simulink model "IndustrialMicrogrid"  (R2025a)
settings: Solver=FixedStepAuto  StartTime=0.0  StopTime=8  FixedStep=Ts  RelTol=1e-3
PostLoadFcn:
  | IndustrialMicrogridInputData
  | GfmGridFormingConverterInputParameters
model workspace (MAT data in the model file):
  caseNum = 2
undefined symbols (not defined in the file): base, BESS, DiscIntNeverNeededParam, grid, Grid, gridInverter, machine, microgrid, PV, PVInverter, PVTransformer, scrFactorRg, scrFactorXg, transformer, Transition_and_Dispatch_ControlModeType, Ts
libraries: ee_lib x126, fl_lib x91, eeGeneralControl x73, nesl_utility x50, nesl_utility_internal x46, simulink x30, eeTransforms x11, eeSinusoidalMeasurementV2 x5, eeTotalHarmonicDistorsion x4, slpidlib x3, simulink_extras x2, eePowerMeasurement x2
(part 2 of 12)

== system IndustrialMicrogrid/MG2 Main Grid ==
  Electrical Reference1 : fl_lib/Electrical/Electrical Elements/Electrical Reference
  Main Grid Frequency : Constant  Value=grid.frequency  SampleTime=-1
  Programmable Voltage Source (Three-Phase)2 : ee_lib/Sources/Programmable Voltage Source (Three-Phase)  magnitude_type=ee.enum.timechanging.constant  vline_rms=grid.voltageSource V  magn_ramp=1 V/s  magn_step=1 V  magn_modu_magn=1 V  magn_modu_freq=1 Hz  magn_t1=1 s  magn_t2=2 s  frequency_type=ee.enum.timechanging.external  freq=50 Hz  freq_ramp=1 Hz/s  freq_step=1 Hz  freq_modu_magn=1 Hz  freq_modu_freq=1 Hz  freq_t1=1 s  freq_t2=2 s  phase_type=ee.enum.timechanging.constant  shift=0 deg  phase_ramp=1 deg/s  phase_step=1 deg  phase_modu_magn=1 deg  phase_modu_freq=1 Hz  phase_t1=1 s  phase_t2=2 s  impedance_option=1  SShortCircuit=100e6 A*V  XR=15  R=0.01 Ohm  L=3.97e-4*0.1 H  G_parasitic=1e-6 1/Ohm  harmonic_option=0  harmonic_orders=[5, 7, 11, 13]  harmonic_ratios=[.1, .1, .1, .1]  harmonic_shifts=[0, 0, 0, 0] deg  harmonic_sequences=[1, 1, 1, 1]  harmonic_t1=-inf s  harmonic_t2=inf s  I_specify=on  I_priority=None  I=[0, 0, 0] A  I_nominal_specify=off  I_nominal_value=1  I_nominal_unit=A  V_specify=on  V_priority=None  V=[0, 0, 0] V  V_nominal_specify=off  V_nominal_value=1  V_nominal_unit=V
      settings: InternalSimscapePortConfiguration="{\"Bottom\":[],\"Left\":[{\"id\":\"ext_freq\",\"label\":\"F\",\"type\":\"input\"},{\"id\":\"n\",\"label\":\"n\",\"type\":\"foundation.electrical.electrical\"}],\"Right\":[{\"id\":\"N\",\"label\":\"~\",\"type\":\"foundation.electrical.three_phase\"}],\"Top\":[]}"
  Simulink-PS Converter : nesl_utility_internal/Simulink-PS Converter  PhysicalDomain=network_engine_domain  SubClassName=ps_input  LeftPortType=input  RightPortType=output  PseudoPeriodic=off  Frequencies=[]  NoiseDistribution=none  NoiseParameters=[]  Unit=1  AffineConversion=off  FilteringAndDerivatives=provide  SimscapeFilterOrder=1  InputFilterTimeConstant=0.001  UdotUserProvided=0
  Source impedance and Line X/R=18.8 : ee_lib/Passive/RLC Assemblies/RLC (Three-Phase)  port_option=ee.enum.threePhasePort.composite  component_structure=ee.enum.rlc.structure.SeriesRL  R=grid.rMV Ohm  L=grid.lMV1 H  C=1e-6 F  R_parasitic=1e-6 Ohm  G_parasitic=1e-6 1/Ohm  IL_specify=on  IL_priority=None  IL=[0, 0, 0] A  IL_nominal_specify=off  IL_nominal_value=1  IL_nominal_unit=A  VC_specify=off  VC_priority=High  VC=[0, 0, 0] V  VC_nominal_specify=off  VC_nominal_value=1  VC_nominal_unit=V
      settings: InternalSimscapePortConfiguration="{\"Bottom\":[],\"Left\":[{\"id\":\"N1\",\"label\":\"~1\",\"type\":\"foundation.electrical.three_phase\"}],\"Right\":[{\"id\":\"N2\",\"label\":\"~2\",\"type\":\"foundation.electrical.three_phase\"}],\"Top\":[]}"
  ref : PMIOPort  Side=Left
  ~ : PMIOPort  Port=2  Side=Right
  wires:
  Main Grid Frequency/1 -> Simulink-PS Converter/1
  connections:
  ref/RConn1 -- Electrical Reference1/LConn1 -- Programmable Voltage Source (Three-Phase)2/LConn2
  Source impedance and Line X/R=18.8/LConn1 -- Programmable Voltage Source (Three-Phase)2/RConn1
  Source impedance and Line X/R=18.8/RConn1 -- ~/RConn1
  Simulink-PS Converter/RConn1 -- Programmable Voltage Source (Three-Phase)2/LConn1

== system IndustrialMicrogrid/MG2 PV Plant ==
  (500KWp PV) : Subsystem
      settings: PortSchema="{\"entries\":[{\"content\":{\"sides\":[{\"content\":{\"connectorIds\":[\"Out1\",\"In1\",\"LConn1\"]},\"type\":\"ConnectorPlacement.EquallySpacedRectSide\",\"uuid\":\"7b0e71bf-88d0-4fd9-b424-51733315768d\"},{\"content\":{\"side\":\"RIGHT\"},\"type\":\"ConnectorPlacement.EquallySpacedRectSide\",\"uuid\":\"454a206f-9a61-4ac7-86a8-f6508f61436e\"},{\"content\":{\"side\":\"TOP\"},\"type\":\"ConnectorPlacement.EquallySpacedRectSide\",\"uuid\":\"cf982e1c-b164-4d0a-abcb-f158cc5498a1\"}]},\"type\":\"ConnectorPlacement.EquallySpacedConnector\",\"uuid\":\"7d6089e9-e0b0-4b95-be20-3597ac4fefae\"}],\"packageUris\":[\"http://schema.mathworks.com/mf0/Connector/R2020b\"],\"version\":\"1.0\"}"
  4.16 kV/ 13.8 kV2 : ee_lib/Passive/Transformers/Two-Winding Transformer (Three-Phase)  SRated=PVTransformer.VA A*V  FRated=grid.frequency Hz  Winding1Connection=ee.enum.windingconnection.delta1  VRated1=PVTransformer.hv V  Winding2Connection=ee.enum.windingconnection.Yn  VRated2=PVTransformer.lv V  CoreType=ee.enum.coretype.threelimb  pu_Rw1=PVTransformer.windingResistance*1/2  pu_Rw2=PVTransformer.windingResistance*1/2  leakage_reactance_option=ee.enum.transformer_leakage.include  pu_Xl1=PVTransformer.windingLekageReactance*1/2  pu_Xl2=PVTransformer.windingLekageReactance*1/2  magnetizing_resistance_option=ee.enum.transformer_magnetizingResistance.exclude  pu_Rm=500  magnetizing_reactance_option=ee.enum.transformer_magnetizingReactance.exclude  saturation_option=ee.enum.transformer_saturation.exclude  pu_Xm=500  current_data=[0, .002, 1, 2]  magnetic_flux_data=[0, 1.2, 1.5, 1.51]  pu_X0=PVTransformer.zeroSequenceReactance*1.5  i1_specify=off  i1_priority=None  i1=[0, 0, 0] A  i1_nominal_specify=off  i1_nominal_value=1  i1_nominal_unit=A  i2_specify=off  i2_priority=None  i2=[0, 0, 0] A  i2_nominal_specify=off  i2_nominal_value=1  i2_nominal_unit=A  phi_specify=off  phi_priority=None  phi=[0, 0, 0]  phi_nominal_specify=off  phi_nominal_value=1  phi_nominal_unit=1  power_dissipated_specify=off  power_dissipated_priority=None  power_dissipated=0 W  power_dissipated_nominal_specify=off  power_dissipated_nominal_value=1  power_dissipated_nominal_unit=W
      settings: InternalSimscapePortConfiguration="{\"Bottom\":[],\"Left\":[{\"id\":\"N1\",\"label\":\"~1\",\"type\":\"foundation.electrical.three_phase\"}],\"Right\":[{\"id\":\"N2\",\"label\":\"~2\",\"type\":\"foundation.electrical.three_phase\"},{\"id\":\"n2\",\"label\":\"n2\",\"type\":\"foundation.electrical.electrical\"}],\"Top\":[]}"
  Bus Creator : BusCreator  Inputs=2
  Bus Selector : BusSelector  OutputSignals=Vmag
  Circuit Breaker : Subsystem
  Current and Voltage Sensor (Three-Phase)1 : ee_lib/Sensors & Transducers/Current and Voltage Sensor (Three-Phase)  vMeasurementType=ee.enum.vmeasurement.lg  outputUnit=ee.enum.unit.pu  SRated=PV.MVABaseNew A*V  VRated=PV.kVBaseNew V  I_specify=off  I_priority=None  I=[0, 0, 0] A  I_nominal_specify=off  I_nominal_value=1  I_nominal_unit=A  V_specify=off  V_priority=None  V=[0, 0, 0] V  V_nominal_specify=off  V_nominal_value=1  V_nominal_unit=V
      settings: InternalSimscapePortConfiguration="{\"Bottom\":[],\"Left\":[{\"id\":\"N1\",\"label\":\"~1\",\"type\":\"foundation.electrical.three_phase\"}],\"Right\":[{\"id\":\"V_output\",\"label\":\"V\",\"type\":\"output\"},{\"id\":\"I_output\",\"label\":\"I\",\"type\":\"output\"},{\"id\":\"N2\",\"label\":\"~2\",\"type\":\"foundation.electrical.three_phase\"}],\"Top\":[]}"
  Electrical Reference8 : fl_lib/Electrical/Electrical Elements/Electrical Reference
  PLL & Measurements2 : Subsystem
  PS-Simulink Converter1 : nesl_utility/PS-Simulink Converter  PhysicalDomain=network_engine_domain  SubClassName=ps_output  LeftPortType=input  RightPortType=output  PseudoPeriodic=off  Frequencies=[]  VectorFormat=inherit  Unit=inherit  AffineConversion=off
  PS-Simulink Converter2 : nesl_utility/PS-Simulink Converter  PhysicalDomain=network_engine_domain  SubClassName=ps_output  LeftPortType=input  RightPortType=output  PseudoPeriodic=off  Frequencies=[]  VectorFormat=inherit  Unit=inherit  AffineConversion=off
  Step : Step  Time=microgrid.controller2PVBrk  Before=1  After=0  SampleTime=2*Ts
  Terminator : Terminator
  ~ : PMIOPort  Side=Left
  mPV : Outport
  wires:
  (500KWp PV)/1(PV) -> Bus Creator/1  "PV"
  PS-Simulink Converter1/1 -> Terminator/1
  Bus Creator/1 -> mPV/1  "mPV"
  PLL & Measurements2/1(Vbus) -> (500KWp PV)/1(Vbus), Bus Selector/1
  PS-Simulink Converter2/1 -> PLL & Measurements2/1(V)
  Bus Selector/1 -> Bus Creator/2  "<Vmag>"
  Step/1 -> Circuit Breaker/1(BRK)
  connections:
  Current and Voltage Sensor (Three-Phase)1/RConn3 -- 4.16 kV/ 13.8 kV2/RConn1
  Current and Voltage Sensor (Three-Phase)1/RConn2 -- PS-Simulink Converter1/LConn1
  4.16 kV/ 13.8 kV2/RConn2 -- Electrical Reference8/LConn1
  Current and Voltage Sensor (Three-Phase)1/RConn1 -- PS-Simulink Converter2/LConn1
  4.16 kV/ 13.8 kV2/LConn1 -- ~/RConn1
  Circuit Breaker/RConn1 -- Current and Voltage Sensor (Three-Phase)1/LConn1
  Circuit Breaker/LConn1 -- (500KWp PV)/LConn1

== system IndustrialMicrogrid/MG2 Power Center ==
  Bus Element In1 : Inport  PortName=ControlRoom  Element=brk2
  Bus Element In2 : Inport  PortName=ControlRoom  Element=dieselBrk
  Bus Element In4 : Inport  PortName=ControlRoom  Element=brk3
  Bus Element In3 : Inport  PortName=ControlRoom  Element=brk1
  BusElementIn : Inport  PortName=ControlRoom  Element=brk4
  Circuit Breaker : Subsystem
  Circuit Breaker1 : Subsystem
      settings: PortSchema="{\"entries\":[{\"content\":{\"sides\":[{\"content\":{\"connectorIds\":[\"LConn1\",\"In1\"]},\"type\":\"ConnectorPlacement.EquallySpacedRectSide\",\"uuid\":\"61e5b689-674d-42bf-9486-b78d237e4dc5\"},{\"content\":{\"connectorIds\":[\"RConn1\"],\"side\":\"RIGHT\"},\"type\":\"ConnectorPlacement.EquallySpacedRectSide\",\"uuid\":\"9e681376-db09-4bc3-bcf5-1ab917668327\"},{\"content\":{\"side\":\"TOP\"},\"type\":\"ConnectorPlacement.EquallySpacedRectSide\",\"uuid\":\"9b4580d8-22f1-4808-acc6-ee968907ce8f\"},{\"content\":{\"side\":\"BOTTOM\"},\"type\":\"ConnectorPlacement.EquallySpacedRectSide\",\"uuid\":\"ecc9f1e9-f021-446f-9399-19e509bfd837\"}]},\"type\":\"ConnectorPlacement.EquallySpacedConnector\",\"uuid\":\"3c8ab3c7-5612-487b-b971-89e63217e257\"}],\"packageUris\":[\"http://schema.mathworks.com/mf0/Connector/R2020b\"],\"version\":\"1.0\"}"
  Circuit Breaker3 : Subsystem
  Circuit Breaker4 : Subsystem
  Diesel Generator : Subsystem
      mask Display: image('$imagefile'); % Use "Edit Image" on toolstrip to change.
  Diesel Measurements : Subsystem
  Fault (Three-Phase) : ee_lib/Utilities/Fault (Three-Phase)  fault_type_option=11  R_pn_fault=3 Ohm  R_ng_fault=3 Ohm  exposemeasurement=ee.enum.exposemeasurement.hidden  enable_external_fault=ee.enum.external_fault.hidden  fault_threshold=0.5  fault_condition=1  fault_resettable=0  enable_temporal_fault=1  fault_start_time=microgrid.controller2PowerCenterFault s  fault_duration=0.3 s  G_parasitic=1e-6 1/Ohm
      settings: InternalSimscapePortConfiguration="{\"Bottom\":[],\"Left\":[{\"id\":\"N\",\"label\":\"~\",\"type\":\"foundation.electrical.three_phase\"}],\"Right\":[],\"Top\":[]}"
  Line X/R=1.44 1 : ee_lib/Passive/RLC Assemblies/RLC (Three-Phase)  port_option=ee.enum.threePhasePort.composite  component_structure=ee.enum.rlc.structure.SeriesRL  R=microgrid.rLine*0.2 Ohm  L=microgrid.lLine*0.2 H  C=1 F  R_parasitic=1e-6 Ohm  G_parasitic=1e-5 1/Ohm  IL_specify=on  IL_priority=None  IL=[0, 0, 0] A  IL_nominal_specify=off  IL_nominal_value=1  IL_nominal_unit=A  VC_specify=on  VC_priority=High  VC=[0, 0, 0] V  VC_nominal_specify=off  VC_nominal_value=1  VC_nominal_unit=V
      settings: InternalSimscapePortConfiguration="{\"Bottom\":[],\"Left\":[{\"id\":\"N1\",\"label\":\"~1\",\"type\":\"foundation.electrical.three_phase\"}],\"Right\":[{\"id\":\"N2\",\"label\":\"~2\",\"type\":\"foundation.electrical.three_phase\"}],\"Top\":[]}"
  Line X/R=1.44 2 : ee_lib/Passive/RLC Assemblies/RLC (Three-Phase)  port_option=ee.enum.threePhasePort.composite  component_structure=ee.enum.rlc.structure.SeriesRL  R=microgrid.rLine*0.3 Ohm  L=microgrid.lLine*0.3 H  C=1 F  R_parasitic=1e-6 Ohm  G_parasitic=1e-5 1/Ohm  IL_specify=on  IL_priority=None  IL=[0, 0, 0] A  IL_nominal_specify=off  IL_nominal_value=1  IL_nominal_unit=A  VC_specify=on  VC_priority=High  VC=[0, 0, 0] V  VC_nominal_specify=off  VC_nominal_value=1  VC_nominal_unit=V
      settings: InternalSimscapePortConfiguration="{\"Bottom\":[],\"Left\":[{\"id\":\"N1\",\"label\":\"~1\",\"type\":\"foundation.electrical.three_phase\"}],\"Right\":[{\"id\":\"N2\",\"label\":\"~2\",\"type\":\"foundation.electrical.three_phase\"}],\"Top\":[]}"
  Line X/R=1.44 3 : ee_lib/Passive/RLC Assemblies/RLC (Three-Phase)  port_option=ee.enum.threePhasePort.composite  component_structure=ee.enum.rlc.structure.SeriesRL  R=microgrid.rLine*0.2 Ohm  L=microgrid.lLine*0.2 H  C=1 F  R_parasitic=1e-6 Ohm  G_parasitic=1e-5 1/Ohm  IL_specify=on  IL_priority=None  IL=[0, 0, 0] A  IL_nominal_specify=off  IL_nominal_value=1  IL_nominal_unit=A  VC_specify=on  VC_priority=High  VC=[0, 0, 0] V  VC_nominal_specify=off  VC_nominal_value=1  VC_nominal_unit=V
      settings: InternalSimscapePortConfiguration="{\"Bottom\":[],\"Left\":[{\"id\":\"N1\",\"label\":\"~1\",\"type\":\"foundation.electrical.three_phase\"}],\"Right\":[{\"id\":\"N2\",\"label\":\"~2\",\"type\":\"foundation.electrical.three_phase\"}],\"Top\":[]}"
  Low-Pass Filter (Discrete or Continuous) : eeGeneralControl/Low-Pass Filter (Discrete or Continuous)  K=1  T=0.1  B=inf  A=-inf  init_option=Inherited from block input  x0=0  Ts=Ts
  Low-Pass Filter (Discrete or Continuous)1 : eeGeneralControl/Low-Pass Filter (Discrete or Continuous)  K=1  T=0.1  B=inf  A=-inf  init_option=Inherited from block input  x0=0  Ts=Ts
  PS-Simulink Converter8 : nesl_utility_internal/PS-Simulink Converter  PhysicalDomain=network_engine_domain  SubClassName=ps_output  LeftPortType=input  RightPortType=output  PseudoPeriodic=off  Frequencies=[]  VectorFormat=1-D array  Unit=MW  AffineConversion=off
  PS-Simulink Converter9 : nesl_utility_internal/PS-Simulink Converter  PhysicalDomain=network_engine_domain  SubClassName=ps_output  LeftPortType=input  RightPortType=output  PseudoPeriodic=off  Frequencies=[]  VectorFormat=1-D array  Unit=MV*A  AffineConversion=off
  Power Sensor (Three-Phase)2 : ee_lib/Sensors & Transducers/Power Sensor (Three-Phase)  load_type=ee.enum.passive.type_balanced.balanced  f0=60 Hz  config=ee.enum.with_neutral.no  rho=1
      settings: InternalSimscapePortConfiguration="{\"Bottom\":[],\"Left\":[{\"id\":\"N1\",\"label\":\"~1\",\"type\":\"foundation.electrical.three_phase\"}],\"Right\":[{\"id\":\"N2\",\"label\":\"~2\",\"type\":\"foundation.electrical.three_phase\"}],\"Top\":[{\"id\":\"Pm\",\"label\":\"P\",\"type\":\"output\"},{\"id\":\"Qm\",\"label\":\"Q\",\"type\":\"output\"}]}"
  Transformer and Disconnectors : Subsystem
      mask Display: image('$imagefile'); % Use "Edit Image" on toolstrip to change.
  Two-Winding Transformer (Three-Phase)1 : ee_lib/Passive/Transformers/Two-Winding Transformer (Three-Phase)  SRated=microgrid.powerCenterTransformerRating A*V  FRated=microgrid.frequency Hz  Winding1Connection=ee.enum.windingconnection.Y  VRated1=microgrid.powerCenterTransformerPrimaryVoltage V  Winding2Connection=ee.enum.windingconnection.Y  VRated2=microgrid.powerCenterTransformerSecondaryVoltage V  CoreType=ee.enum.coretype.threelimb  pu_Rw1=microgrid.powerCenterPrimaryresistance  pu_Rw2=microgrid.powerCenterPrimaryreactance  leakage_reactance_option=ee.enum.transformer_leakage.include  pu_Xl1=microgrid.powerCenterSecondaryresistance  pu_Xl2=microgrid.powerCenterSecondaryreactance  magnetizing_resistance_option=ee.enum.transformer_magnetizingResistance.include  pu_Rm=500  magnetizing_reactance_option=ee.enum.transformer_magnetizingReactance.include  saturation_option=ee.enum.transformer_saturation.exclude  pu_Xm=500  current_data=[0, .002, 1, 2]  magnetic_flux_data=[0, 1.2, 1.5, 1.51]  pu_X0=0.5  i1_specify=on  i1_priority=None  i1=[0, 0, 0] A  i1_nominal_specify=off  i1_nominal_value=1  i1_nominal_unit=A  i2_specify=on  i2_priority=None  i2=[0, 0, 0] A  i2_nominal_specify=off  i2_nominal_value=1  i2_nominal_unit=A  phi_specify=off  phi_priority=None  phi=[0, 0, 0]  phi_nominal_specify=off  phi_nominal_value=1  phi_nominal_unit=1  power_dissipated_specify=off  power_dissipated_priority=None  power_dissipated=0 W  power_dissipated_nominal_specify=off  power_dissipated_nominal_value=1  power_dissipated_nominal_unit=W
      settings: InternalSimscapePortConfiguration="{\"Bottom\":[],\"Left\":[{\"id\":\"N1\",\"label\":\"~1\",\"type\":\"foundation.electrical.three_phase\"}],\"Right\":[{\"id\":\"N2\",\"label\":\"~2\",\"type\":\"foundation.electrical.three_phase\"}],\"Top\":[]}"
  Conn2 : PMIOPort  Side=Left
  ~ a : PMIOPort  Port=2  Side=Left
  " ~ " : PMIOPort  Port=3  Side=Right
  Out Bus Element2 : Outport  PortName=mPowerCentre  Element=tieline.activepower
  Out Bus Element3 : Outport  PortName=mPowerCentre  Element=tieline.reactivepower
  Out Bus Element1 : Outport  PortName=mPowerCentre  Element=diesel
  wires:
  Bus Element In3/1 -> Circuit Breaker/1(BRK)
  PS-Simulink Converter8/1 -> Low-Pass Filter (Discrete or Continuous)/1
  Low-Pass Filter (Discrete or Continuous)1/1 -> Out Bus Element3/1
  PS-Simulink Converter9/1 -> Low-Pass Filter (Discrete or Continuous)1/1
  Low-Pass Filter (Discrete or Continuous)/1 -> Out Bus Element2/1
  Bus Element In4/1 -> Circuit Breaker3/1(BRK)
  Bus Element In2/1 -> Circuit Breaker4/1(BRK)
  Diesel Measurements/1(mdiesel) -> Out Bus Element1/1  "diesel"
  Bus Element In1/1 -> Circuit Breaker1/1(BRK)
  BusElementIn/1 -> Transformer and Disconnectors/1(BRK)
  connections:
  Line X/R=1.44 1/RConn1 -- ~ a/RConn1 -- Fault (Three-Phase)/LConn1
  Line X/R=1.44 3/RConn1 -- " ~ "/RConn1
  Circuit Breaker/RConn1 -- Circuit Breaker3/LConn1 -- Circuit Breaker1/LConn1
  Line X/R=1.44 2/LConn1 -- Conn2/RConn1
  Diesel Generator/RConn1 -- Transformer and Disconnectors/LConn1
  Two-Winding Transformer (Three-Phase)1/RConn1 -- Circuit Breaker4/RConn1 -- Line X/R=1.44 3/LConn1
  Transformer and Disconnectors/RConn1 -- Diesel Measurements/LConn1
  Circuit Breaker3/RConn1 -- Line X/R=1.44 1/LConn1
  PS-Simulink Converter9/LConn1 -- Power Sensor (Three-Phase)2/LConn3
  PS-Simulink Converter8/LConn1 -- Power Sensor (Three-Phase)2/LConn2
  Power Sensor (Three-Phase)2/LConn1 -- Line X/R=1.44 2/RConn1
  Circuit Breaker/LConn1 -- Power Sensor (Three-Phase)2/RConn1
  Circuit Breaker1/RConn1 -- Two-Winding Transformer (Three-Phase)1/LConn1
  Circuit Breaker4/LConn1 -- Diesel Measurements/RConn1

== system IndustrialMicrogrid/MG2 Primary Substation ==
  ControlRoom : Inport
  BESS and Controller : Subsystem
  Bus Selector : BusSelector  OutputSignals=Substation.brk
  Circuit Breaker : Subsystem
  Microgrid Controller : Subsystem  mask{resynchronization=on, plannedIslanding=on, blackStart=on, kpPLL=microgrid.KpPLLController2, kiPLL=microgrid.KiPLLController2, frequencyPLL=grid.frequency, sampleTimePLL=Ts, pUpperLimit=1.2, pLowerLimit=-1.2, qUpperLimit=1.2, qLowerLimit=-1.2, gridFrequency=grid.frequency, resyncDelay=microgrid.resynchDelay, kpVoltage=microgrid.KpVolResynch2, kiVoltage=microgrid.KiVolResynch2, voltageThreshold=microgrid.voltageThreshold, voltageDroop=microgrid.KDroop, kpFrequency=microgrid.KpFreResynch2, kiFrequency=microgrid.KiFreResynch2, frequencyThreshold=microgrid.frequencyThreshold, kpAngle=microgrid.KpAngResynch2, kiAngle=microgrid.KiAngResynch2, angleThreshold=microgrid.angleThreshold, plannedIslandingDelay=microgrid.plannedIslandDelay, kpActive=microgrid.KpPPlannedIsland2, kiActive=microgrid.KiPPlannedIsland2, activeThreshold=microgrid.zeroActivePowerThreshold, kpReactive=microgrid.KpQPlannedIsland2, kiReactive=microgrid.KiQPlannedIsland2, reactiveThreshold=microgrid.zeroReactivePowerThreshold, blackStartTime=microgrid.controller2BlackStartDelay, blackStartFrequency=60, level1=microgrid.controller2BlackStartVoltageLevel1, level2=microgrid.controller2BlackStartVoltageLevel2, level3=microgrid.controller2BlackStartVoltageLevel3, delay1=microgrid.controller2BlackStartDelayLevel1, delay2=microgrid.controller2BlackStartDelayLevel2, delay3=microgrid.controller2BlackStartDelayLevel3, upperVoltagelimit=1.1, lowerVoltageLimit=0.9, upperFrequencyLimit=60.6, lowerFrequencyLimit=59.4}
      mask prompts: plannedIslanding "Planned Islanding"; blackStart "Black Start"; kpPLL "Proportional Gain"; kiPLL "Integral Gain"; frequencyPLL "Grid Frequency in Hz"; sampleTimePLL "Sample Time in sec"; pUpperLimit "Upper Limit in pu"; pLowerLimit "Lower Limit in pu"; qUpperLimit "Upper Limit in pu"; qLowerLimit "Lower Limit in pu"; gridFrequency "Grid Frequency in Hz"; resyncDelay "Delay in sec"; kpVoltage "Proportional Gain"; kiVoltage "Voltage Integral Gain"; voltageThreshold "Threshold"; voltageDroop "Reactive Power Droop"; kpFrequency "Proportional Gain"; kiFrequency "Integral Gain"; frequencyThreshold "Threshold"; kpAngle "Proportional Gain"; kiAngle "Integral Gain"; angleThreshold "Threshold"; plannedIslandingDelay "Delay in sec"; kpActive "Proportional Gain"; kiActive "Integral Gain"; activeThreshold "Threshold"; kpReactive "Proportional Gain"; kiReactive "Integral Gain"; reactiveThreshold "Threshold"; blackStartTime "Black Start Time in sec"; blackStartFrequency "Reference Frequency in Hz"; level1 "Level 1 in pu"; level2 "Level 2 in pu"; level3 "Level 3 in pu"; delay1 "Delay 1 in sec"; delay2 "Delay2 in sec"; delay3 "Delay3 in sec"; upperVoltagelimit "Maximum Voltage in pu"; lowerVoltageLimit "Minimum Voltage in pu"; upperFrequencyLimit "Maximum frequency in Hz"; lowerFrequencyLimit "Minimum Frequency in Hz"
      mask init: same as IndustrialMicrogrid/MG1 Primary Substation/Microgrid Controller
      mask Callback resynchronization:
      | plannedIslandingBlock = [gcb,'/','Microgrid Control Functions','/','Planned Islanding'];
      | resynchBlock = [gcb,'/','Microgrid Control Functions','/','Resynchronization'];
      | blackStartBlock = [gcb,'/','Microgrid Control Functions','/','Black Start'];
      | block = {resynchBlock,plannedIslandingBlock,blackStartBlock};
      | blockEnable = {get_param(gcb,'resynchronization'),get_param(gcb,'plannedIslanding'),get_param(gcb,'blackStart')};
      | parameterIdx = {12:23,24:30,31:38};
      | % Set the 'MaskVisibilities' property for each parameters
      | cArray=cell(1,42);
      | cArray(:)={'on'};
      | for blockIdx = 1:length(block)
      |     if strcmp(blockEnable{blockIdx},'on')
      |         cArray(parameterIdx{blockIdx}) = {'on'};
      |     else
      |         cArray(parameterIdx{blockIdx}) = {'off'};
      |     end
      | end
      | set_param(gcb,'MaskVisibilities',cArray);
      mask Callback plannedIslanding:
      | plannedIslandingBlock = [gcb,'/','Microgrid Control Functions','/','Planned Islanding'];
      | resynchBlock = [gcb,'/','Microgrid Control Functions','/','Resynchronization'];
      | blackStartBlock = [gcb,'/','Microgrid Control Functions','/','Black Start'];
      | block = {resynchBlock,plannedIslandingBlock,blackStartBlock};
      | blockEnable = {get_param(gcb,'resynchronization'),get_param(gcb,'plannedIslanding'),get_param(gcb,'blackStart')};
      | parameterIdx = {12:23,24:30,31:38};
      | % Set the 'MaskVisibilities' property for each parameters
      | cArray=cell(1,42);
      | cArray(:)={'on'};
      | for blockIdx = 1:length(block)
      |     if strcmp(blockEnable{blockIdx},'on')
      |         cArray(parameterIdx{blockIdx}) = {'on'};
      |     else
      |         cArray(parameterIdx{blockIdx}) = {'off'};
      |     end
      | end
      | set_param(gcb,'MaskVisibilities',cArray);
      mask Callback blackStart:
      | plannedIslandingBlock = [gcb,'/','Microgrid Control Functions','/','Planned Islanding'];
      | resynchBlock = [gcb,'/','Microgrid Control Functions','/','Resynchronization'];
      | blackStartBlock = [gcb,'/','Microgrid Control Functions','/','Black Start'];
      | block = {resynchBlock,plannedIslandingBlock,blackStartBlock};
      | blockEnable = {get_param(gcb,'resynchronization'),get_param(gcb,'plannedIslanding'),get_param(gcb,'blackStart')};
      | parameterIdx = {12:23,24:30,31:38};
      | % Set the 'MaskVisibilities' property for each parameters
      | cArray=cell(1,42);
      | cArray(:)={'on'};
      | for blockIdx = 1:length(block)
      |     if strcmp(blockEnable{blockIdx},'on')
      |         cArray(parameterIdx{blockIdx}) = {'on'};
      |     else
      |         cArray(parameterIdx{blockIdx}) = {'off'};
      |     end
      | end
      | set_param(gcb,'MaskVisibilities',cArray);
      mask DialogControl ParameterGroupVar Prompt: Microgrid control functions
      mask DialogControl Container22 Prompt: PLL
      mask DialogControl Container25 Prompt: General
      mask DialogControl Container23 Prompt: Reference Generation
      mask DialogControl Container27 Prompt: Active Power
      mask DialogControl Container28 Prompt: Reactive Power
      mask DialogControl Container3 Prompt: Resynchronization
      mask DialogControl Container15 Prompt: General
      mask DialogControl Container9 Prompt: Voltage
      mask DialogControl Container10 Prompt: Frequency
      mask DialogControl Container11 Prompt: Angle
      mask DialogControl Container8 Prompt: Planned Islanding
      mask DialogControl Container16 Prompt: General
      mask DialogControl Container13 Prompt: Active Power
      mask DialogControl Container14 Prompt: Reactive Power
      mask DialogControl Container17 Prompt: Black Start
      mask DialogControl Container19 Prompt: General
      mask DialogControl Container20 Prompt: Voltage Levels
      mask DialogControl Container21 Prompt: Time Delays
      mask DialogControl Container261 Prompt: Power Quality Metrics
      mask Display: image('$imagefile'); % Use "Edit Image" on toolstrip to change.
  PCC Measurements and PCC Breaker : Subsystem
      settings: PortSchema="{\"entries\":[{\"content\":{\"sides\":[{\"content\":{\"connectorIds\":[\"In1\",\"LConn1\"]},\"type\":\"ConnectorPlacement.EquallySpacedRectSide\",\"uuid\":\"8d1da80d-0887-44e0-a470-a36b233902dd\"},{\"content\":{\"connectorIds\":[\"RConn1\",\"Out1\"],\"side\":\"RIGHT\"},\"type\":\"ConnectorPlacement.EquallySpacedRectSide\",\"uuid\":\"69fb492f-8375-4103-b8b2-15eabe039e82\"},{\"content\":{\"side\":\"TOP\"},\"type\":\"ConnectorPlacement.EquallySpacedRectSide\",\"uuid\":\"e2b1d5d4-ee63-40b0-8f64-d550ce16e67b\"}]},\"type\":\"ConnectorPlacement.EquallySpacedConnector\",\"uuid\":\"58949bb1-e57a-47d5-a7ba-dffc622c6db7\"}],\"packageUris\":[\"http://schema.mathworks.com/mf0/Connector/R2020b\"],\"version\":\"1.0\"}"
      mask Display: image('$imagefile'); % Use "Edit Image" on toolstrip to change.
  Transformer and Disconnectors : Subsystem
      mask Display: image('$imagefile'); % Use "Edit Image" on toolstrip to change.
  ~ : PMIOPort  Side=Left
  "~ " : PMIOPort  Port=2  Side=Right
  Out Bus Element : Outport  PortName=MG2  Element=mBESS
  Out Bus Element1 : Outport  PortName=MG2  Element=mPCC
  Out Bus Element2 : Outport  PortName=MG2  Element=MGController
  wires:
  ControlRoom/1 -> BESS and Controller/1(CntrlRmIN), Bus Selector/1, Microgrid Controller/1(CtrlRm)
  Microgrid Controller/3(PQRef) -> BESS and Controller/4(PQref)
  Microgrid Controller/2(FRef) -> BESS and Controller/3(f0)
  Microgrid Controller/1(VRef) -> BESS and Controller/2(Vref)
  Microgrid Controller/5(PCC BRK) -> PCC Measurements and PCC Breaker/1(cBreaker)
  PCC Measurements and PCC Breaker/1(" mPCC") -> Out Bus Element1/1, Microgrid Controller/2(mPCC)  "mPCC"
  BESS and Controller/1(mBESS) -> Out Bus Element/1  "BESS2"
  Microgrid Controller/4(MGController) -> Out Bus Element2/1  "MGController"
  Bus Selector/1 -> Circuit Breaker/1(BRK)  "<brk>"
  connections:
  ~/RConn1 -- Transformer and Disconnectors/LConn1
  Transformer and Disconnectors/RConn1 -- PCC Measurements and PCC Breaker/LConn1
  PCC Measurements and PCC Breaker/RConn1 -- Circuit Breaker/LConn1 -- BESS and Controller/LConn1
  Circuit Breaker/RConn1 -- "~ "/RConn1

== system IndustrialMicrogrid/MG2 Processing, Lighting and Auxiliary Loads ==
  Bus Element In1 : Inport  PortName=ControlRoom  Element=Load3
  Bus Element In4 : Inport  PortName=ControlRoom  Element=Load5
  Bus Element In3 : Inport  PortName=ControlRoom  Element=Load4a
  Bus Element In2 : Inport  PortName=ControlRoom  Element=Load4b
  Circuit Breaker1 : Subsystem
  Circuit Breaker2 : Subsystem
  Circuit Breaker3 : Subsystem
  Circuit Breaker4 : Subsystem
  Electrical Reference1 : fl_lib/Electrical/Electrical Elements/Electrical Reference
  Electrical Reference2 : fl_lib/Electrical/Electrical Elements/Electrical Reference
  Electrical Reference5 : fl_lib/Electrical/Electrical Elements/Electrical Reference
  Load Measurements1 : Subsystem
      settings: PortSchema="{\"entries\":[{\"content\":{\"sides\":[{\"content\":{\"connectorIds\":[\"LConn1\"]},\"type\":\"ConnectorPlacement.EquallySpacedRectSide\",\"uuid\":\"d870a913-f96e-493f-ac0f-f00d694ce040\"},{\"content\":{\"connectorIds\":[\"Out1\"],\"side\":\"RIGHT\"},\"type\":\"ConnectorPlacement.EquallySpacedRectSide\",\"uuid\":\"12eea89c-1ef8-4155-8c58-3c970c5d9b18\"},{\"content\":{\"connectorIds\":[],\"side\":\"TOP\"},\"type\":\"ConnectorPlacement.EquallySpacedRectSide\",\"uuid\":\"8c8b4bd0-9ee8-4a98-bcb2-09acde5bae56\"},{\"content\":{\"connectorIds\":[\"RConn1\"],\"side\":\"BOTTOM\"},\"type\":\"ConnectorPlacement.EquallySpacedRectSide\",\"uuid\":\"443bcb6e-ffa1-4f95-8c19-122149ac17cf\"}]},\"type\":\"ConnectorPlacement.EquallySpacedConnector\",\"uuid\":\"4cf8469f-5e58-4383-9537-851b6a4abf90\"}],\"packageUris\":[\"http://schema.mathworks.com/mf0/Connector/R2020b\"],\"version\":\"1.0\"}"
  Load for auxiliary : ee_lib/Passive/RLC Assemblies/Wye-Connected Load  port_option=ee.enum.threePhasePort.composite  parameterization=ee.enum.rlc.parameterization.ratedpower  component_structure=ee.enum.rlc.structure.C  component_structure_PQ=ee.enum.rlc.structure.SeriesRL  R=1 Ohm  L=0.001 H  C=1e-6 F  VRated=microgrid.powerCenterVoltage V  FRated=microgrid.frequency Hz  P=microgrid.pLoad22 W  Qpos=microgrid.qLoad22 A*V  Qneg=-3000 A*V  R_parasitic=1e-6 Ohm  G_parasitic=1e-6 1/Ohm  R_parasitic_PQ=1e-6 Ohm  G_parasitic_PQ=1e-6 1/Ohm  Vmag0=0 V  Vang0=0 deg  Freq0=microgrid.frequency Hz  IL_specify=on  IL_priority=High  IL=[ 0 0 0 ] A  IL_nominal_specify=off  IL_nominal_value=1  IL_nominal_unit=A  VC_specify=on  VC_priority=High  VC=[ 0 0 0 ] V  VC_nominal_specify=off  VC_nominal_value=1  VC_nominal_unit=V
  Load for auxiliary1 : ee_lib/Passive/RLC Assemblies/Wye-Connected Load  port_option=ee.enum.threePhasePort.composite  parameterization=ee.enum.rlc.parameterization.ratedpower  component_structure=ee.enum.rlc.structure.C  component_structure_PQ=ee.enum.rlc.structure.SeriesRL  R=1 Ohm  L=0.001 H  C=1e-6 F  VRated=microgrid.powerCenterVoltage V  FRated=microgrid.frequency Hz  P=microgrid.pLoad33 W  Qpos=microgrid.qLoad33 A*V  Qneg=-3000 A*V  R_parasitic=1e-6 Ohm  G_parasitic=1e-6 1/Ohm  R_parasitic_PQ=1e-6 Ohm  G_parasitic_PQ=1e-6 1/Ohm  Vmag0=0 V  Vang0=0 deg  Freq0=microgrid.frequency Hz  IL_specify=on  IL_priority=High  IL=[ 0 0 0 ] A  IL_nominal_specify=off  IL_nominal_value=1  IL_nominal_unit=A  VC_specify=on  VC_priority=High  VC=[ 0 0 0 ] V  VC_nominal_specify=off  VC_nominal_value=1  VC_nominal_unit=V
  Load for lights : ee_lib/Passive/RLC Assemblies/Wye-Connected Load  port_option=ee.enum.threePhasePort.composite  parameterization=ee.enum.rlc.parameterization.ratedpower  component_structure=ee.enum.rlc.structure.C  component_structure_PQ=ee.enum.rlc.structure.SeriesRL  R=1 Ohm  L=0.001 H  C=1e-6 F  VRated=microgrid.powerCenterVoltage V  FRated=microgrid.frequency Hz  P=microgrid.pLoad21 W  Qpos=microgrid.qLoad21 A*V  Qneg=-3000 A*V  R_parasitic=1e-6 Ohm  G_parasitic=1e-6 1/Ohm  R_parasitic_PQ=1e-6 Ohm  G_parasitic_PQ=1e-6 1/Ohm  Vmag0=0 V  Vang0=0 deg  Freq0=microgrid.frequency Hz  IL_specify=on  IL_priority=High  IL=[ 0 0 0 ] A  IL_nominal_specify=off  IL_nominal_value=1  IL_nominal_unit=A  VC_specify=on  VC_priority=High  VC=[ 0 0 0 ] V  VC_nominal_specify=off  VC_nominal_value=1  VC_nominal_unit=V
  Motor Loads : Subsystem
  RLC (Three-Phase) : ee_lib/Passive/RLC Assemblies/RLC (Three-Phase)  port_option=ee.enum.threePhasePort.composite  component_structure=ee.enum.rlc.structure.SeriesRL  R=1+0.3461 Ohm  L=5e-3+0.0073 H  C=1e-6 F  R_parasitic=0 Ohm  G_parasitic=0 1/Ohm  IL_specify=on  IL_priority=None  IL=[0, 0, 0] A  IL_nominal_specify=off  IL_nominal_value=1  IL_nominal_unit=A  VC_specify=off  VC_priority=High  VC=[0, 0, 0] V  VC_nominal_specify=off  VC_nominal_value=1  VC_nominal_unit=V
      settings: InternalSimscapePortConfiguration="{\"Bottom\":[],\"Left\":[{\"id\":\"N1\",\"label\":\"~1\",\"type\":\"foundation.electrical.three_phase\"}],\"Right\":[{\"id\":\"N2\",\"label\":\"~2\",\"type\":\"foundation.electrical.three_phase\"}],\"Top\":[]}"
  ~ : PMIOPort  Side=Left
  mLoad2 : Outport
  wires:
  Load Measurements1/1(mLoad2) -> mLoad2/1
  Bus Element In1/1 -> Circuit Breaker3/1(BRK)
  Bus Element In2/1 -> Circuit Breaker4/1(BRK)
  Bus Element In3/1 -> Circuit Breaker2/1(BRK)
  Bus Element In4/1 -> Circuit Breaker1/1(BRK)
  connections:
  Electrical Reference2/LConn1 -- Load for lights/RConn1
  ~/RConn1 -- Load Measurements1/LConn1
  Circuit Breaker3/RConn1 -- Load for lights/LConn1
  Circuit Breaker2/RConn1 -- Load for auxiliary/LConn1
  Load for auxiliary/RConn1 -- Electrical Reference5/LConn1
  Load for auxiliary1/RConn1 -- Electrical Reference1/LConn1
  Circuit Breaker4/RConn1 -- Load for auxiliary1/LConn1
  Load Measurements1/RConn1 -- Circuit Breaker3/LConn1 -- Circuit Breaker1/LConn1 -- Circuit Breaker4/LConn1 -- Circuit Breaker2/LConn1
  Circuit Breaker1/RConn1 -- RLC (Three-Phase)/LConn1
  Motor Loads/RConn1 -- RLC (Three-Phase)/RConn1

== system IndustrialMicrogrid/Operator Room ==
  mLoad : Inport
  MGController1 : Inport  Port=2
  mTieline : Inport  Port=3
  MGController2 : Inport  Port=4
  mPV : Inport  Port=5
  mPowerCenter : Inport  Port=6
  mLoad2 : Inport  Port=7
  mLoad3 : Inport  Port=8
  MG1 : Subsystem  Commented=on
  MG2 : Subsystem
  Control Room MG2 : Outport
  Visualization MG1 : Outport  Port=2
  Visualization MG2 : Outport  Port=3
  Control Room MG1 : Outport  Port=4
  wires:
  MGController2/1 -> MG2/1(MG2)  "MGController2"
  mLoad2/1 -> MG2/3(mLoad2)  "mLoad2"
  mPV/1 -> MG2/2(mPV)  "mPV"
  mPowerCenter/1 -> MG2/4(mPowerCentre)  "mPowerCentre"
  MGController1/1 -> MG1/1(MG1)  "MGController1"
  mTieline/1 -> MG1/4(mTieine)  "mTieline"
  MG2/2(Control Room MG2) -> Control Room MG2/1
  MG1/1(Control Room MG1) -> Control Room MG1/1
  MG1/2(Visualization MG1) -> Visualization MG1/1
  MG2/1(Visualization MG2) -> Visualization MG2/1
  mLoad3/1 -> MG1/3(mLoad3)  "mLoad3"
  mLoad/1 -> MG1/2(mLoad)  "mLoad"

== system IndustrialMicrogrid/Selected Results ==
  Input : Inport
  Input1 : Inport  Port=2
  MG1 : Subsystem  Commented=on
  MG2 : Subsystem
  wires:
  Input/1 -> MG1/1(Visualization1)
  Input1/1 -> MG2/1(Visualization)

== system IndustrialMicrogrid/MG1 Drilling Loads/Circuit Breaker1 ==
  BRK : Inport
  Data Type Conversion : DataTypeConversion  OutDataTypeStr=double  SaturateOnIntegerOverflow=off  RndMeth=Floor
  Open Resistance : Gain  Gain=1e5
  Phase Splitter : ee_lib/Connectors & References/Phase Splitter
  Phase Splitter1 : ee_lib/Connectors & References/Phase Splitter
  Simulink-PS Converter : nesl_utility/Simulink-PS Converter  PhysicalDomain=network_engine_domain  SubClassName=ps_input  LeftPortType=input  RightPortType=output  PseudoPeriodic=off  Frequencies=[]  NoiseDistribution=none  NoiseParameters=[]  Unit=1  AffineConversion=off  FilteringAndDerivatives=provide  SimscapeFilterOrder=1  InputFilterTimeConstant=0.001  UdotUserProvided=0
  Variable Resistor : fl_lib/Electrical/Electrical Elements/Variable Resistor  Rmin=1e-3 Ohm  thermalEnable=false  thermal_mass=1 J/K  i_specify=off  i_priority=None  i=0 A  i_nominal_specify=off  i_nominal_value=1  i_nominal_unit=A  v_specify=off  v_priority=None  v=0 V  v_nominal_specify=off  v_nominal_value=1  v_nominal_unit=V  T_specify=off  T_priority=None  T=300 K  T_nominal_specify=off  T_nominal_value=1  T_nominal_unit=K
  Variable Resistor1 : fl_lib/Electrical/Electrical Elements/Variable Resistor  Rmin=1e-3 Ohm  thermalEnable=false  thermal_mass=1 J/K  i_specify=off  i_priority=None  i=0 A  i_nominal_specify=off  i_nominal_value=1  i_nominal_unit=A  v_specify=off  v_priority=None  v=0 V  v_nominal_specify=off  v_nominal_value=1  v_nominal_unit=V  T_specify=off  T_priority=None  T=300 K  T_nominal_specify=off  T_nominal_value=1  T_nominal_unit=K
  Variable Resistor2 : fl_lib/Electrical/Electrical Elements/Variable Resistor  Rmin=1e-3 Ohm  thermalEnable=false  thermal_mass=1 J/K  i_specify=off  i_priority=None  i=0 A  i_nominal_specify=off  i_nominal_value=1  i_nominal_unit=A  v_specify=off  v_priority=None  v=0 V  v_nominal_specify=off  v_nominal_value=1  v_nominal_unit=V  T_specify=off  T_priority=None  T=300 K  T_nominal_specify=off  T_nominal_value=1  T_nominal_unit=K
  In : PMIOPort  Side=Left
  ~ : PMIOPort  Port=2  Side=Right
  wires:
  Data Type Conversion/1 -> Open Resistance/1
  BRK/1 -> Data Type Conversion/1
  Open Resistance/1 -> Simulink-PS Converter/1
  connections:
  Phase Splitter1/RConn2 -- Variable Resistor1/RConn1
  Variable Resistor1/LConn2 -- Phase Splitter/RConn2
  Phase Splitter1/RConn3 -- Variable Resistor2/RConn1
  Phase Splitter/RConn1 -- Variable Resistor/LConn2
  Variable Resistor2/LConn2 -- Phase Splitter/RConn3
  Phase Splitter1/RConn1 -- Variable Resistor/RConn1
  Phase Splitter1/LConn1 -- ~/RConn1
  Variable Resistor/LConn1 -- Simulink-PS Converter/RConn1 -- Variable Resistor2/LConn1 -- Variable Resistor1/LConn1
  Phase Splitter/LConn1 -- In/RConn1

== system IndustrialMicrogrid/MG1 Drilling Loads/Circuit Breaker2 ==
  BRK : Inport
  Data Type Conversion : DataTypeConversion  OutDataTypeStr=double  SaturateOnIntegerOverflow=off  RndMeth=Floor
  Open Resistance : Gain  Gain=1e5
  Phase Splitter : ee_lib/Connectors & References/Phase Splitter
  Phase Splitter1 : ee_lib/Connectors & References/Phase Splitter
  Simulink-PS Converter : nesl_utility/Simulink-PS Converter  PhysicalDomain=network_engine_domain  SubClassName=ps_input  LeftPortType=input  RightPortType=output  PseudoPeriodic=off  Frequencies=[]  NoiseDistribution=none  NoiseParameters=[]  Unit=1  AffineConversion=off  FilteringAndDerivatives=provide  SimscapeFilterOrder=1  InputFilterTimeConstant=0.001  UdotUserProvided=0
  Variable Resistor : fl_lib/Electrical/Electrical Elements/Variable Resistor  Rmin=1e-3 Ohm  thermalEnable=false  thermal_mass=1 J/K  i_specify=off  i_priority=None  i=0 A  i_nominal_specify=off  i_nominal_value=1  i_nominal_unit=A  v_specify=off  v_priority=None  v=0 V  v_nominal_specify=off  v_nominal_value=1  v_nominal_unit=V  T_specify=off  T_priority=None  T=300 K  T_nominal_specify=off  T_nominal_value=1  T_nominal_unit=K
  Variable Resistor1 : fl_lib/Electrical/Electrical Elements/Variable Resistor  Rmin=1e-3 Ohm  thermalEnable=false  thermal_mass=1 J/K  i_specify=off  i_priority=None  i=0 A  i_nominal_specify=off  i_nominal_value=1  i_nominal_unit=A  v_specify=off  v_priority=None  v=0 V  v_nominal_specify=off  v_nominal_value=1  v_nominal_unit=V  T_specify=off  T_priority=None  T=300 K  T_nominal_specify=off  T_nominal_value=1  T_nominal_unit=K
  Variable Resistor2 : fl_lib/Electrical/Electrical Elements/Variable Resistor  Rmin=1e-3 Ohm  thermalEnable=false  thermal_mass=1 J/K  i_specify=off  i_priority=None  i=0 A  i_nominal_specify=off  i_nominal_value=1  i_nominal_unit=A  v_specify=off  v_priority=None  v=0 V  v_nominal_specify=off  v_nominal_value=1  v_nominal_unit=V  T_specify=off  T_priority=None  T=300 K  T_nominal_specify=off  T_nominal_value=1  T_nominal_unit=K
  In : PMIOPort  Side=Left
  ~ : PMIOPort  Port=2  Side=Right
  wires:
  Data Type Conversion/1 -> Open Resistance/1
  BRK/1 -> Data Type Conversion/1
  Open Resistance/1 -> Simulink-PS Converter/1
  connections:
  Phase Splitter1/RConn2 -- Variable Resistor1/RConn1
  Variable Resistor1/LConn2 -- Phase Splitter/RConn2
  Phase Splitter1/RConn3 -- Variable Resistor2/RConn1
  Phase Splitter/RConn1 -- Variable Resistor/LConn2
  Variable Resistor2/LConn2 -- Phase Splitter/RConn3
  Phase Splitter1/RConn1 -- Variable Resistor/RConn1
  Phase Splitter1/LConn1 -- ~/RConn1
  Variable Resistor/LConn1 -- Simulink-PS Converter/RConn1 -- Variable Resistor2/LConn1 -- Variable Resistor1/LConn1
  Phase Splitter/LConn1 -- In/RConn1

== system IndustrialMicrogrid/MG1 Drilling Loads/Circuit Breaker3 ==
  BRK : Inport
  Data Type Conversion : DataTypeConversion  OutDataTypeStr=double  SaturateOnIntegerOverflow=off  RndMeth=Floor
  Open Resistance : Gain  Gain=1e5
  Phase Splitter : ee_lib/Connectors & References/Phase Splitter
  Phase Splitter1 : ee_lib/Connectors & References/Phase Splitter
  Simulink-PS Converter : nesl_utility/Simulink-PS Converter  PhysicalDomain=network_engine_domain  SubClassName=ps_input  LeftPortType=input  RightPortType=output  PseudoPeriodic=off  Frequencies=[]  NoiseDistribution=none  NoiseParameters=[]  Unit=1  AffineConversion=off  FilteringAndDerivatives=provide  SimscapeFilterOrder=1  InputFilterTimeConstant=0.001  UdotUserProvided=0
  Variable Resistor : fl_lib/Electrical/Electrical Elements/Variable Resistor  Rmin=1e-3 Ohm  thermalEnable=false  thermal_mass=1 J/K  i_specify=off  i_priority=None  i=0 A  i_nominal_specify=off  i_nominal_value=1  i_nominal_unit=A  v_specify=off  v_priority=None  v=0 V  v_nominal_specify=off  v_nominal_value=1  v_nominal_unit=V  T_specify=off  T_priority=None  T=300 K  T_nominal_specify=off  T_nominal_value=1  T_nominal_unit=K
  Variable Resistor1 : fl_lib/Electrical/Electrical Elements/Variable Resistor  Rmin=1e-3 Ohm  thermalEnable=false  thermal_mass=1 J/K  i_specify=off  i_priority=None  i=0 A  i_nominal_specify=off  i_nominal_value=1  i_nominal_unit=A  v_specify=off  v_priority=None  v=0 V  v_nominal_specify=off  v_nominal_value=1  v_nominal_unit=V  T_specify=off  T_priority=None  T=300 K  T_nominal_specify=off  T_nominal_value=1  T_nominal_unit=K
  Variable Resistor2 : fl_lib/Electrical/Electrical Elements/Variable Resistor  Rmin=1e-3 Ohm  thermalEnable=false  thermal_mass=1 J/K  i_specify=off  i_priority=None  i=0 A  i_nominal_specify=off  i_nominal_value=1  i_nominal_unit=A  v_specify=off  v_priority=None  v=0 V  v_nominal_specify=off  v_nominal_value=1  v_nominal_unit=V  T_specify=off  T_priority=None  T=300 K  T_nominal_specify=off  T_nominal_value=1  T_nominal_unit=K
  In : PMIOPort  Side=Left
  ~ : PMIOPort  Port=2  Side=Right
  wires:
  Data Type Conversion/1 -> Open Resistance/1
  BRK/1 -> Data Type Conversion/1
  Open Resistance/1 -> Simulink-PS Converter/1
  connections:
  Phase Splitter1/RConn2 -- Variable Resistor1/RConn1
  Variable Resistor1/LConn2 -- Phase Splitter/RConn2
  Phase Splitter1/RConn3 -- Variable Resistor2/RConn1
  Phase Splitter/RConn1 -- Variable Resistor/LConn2
  Variable Resistor2/LConn2 -- Phase Splitter/RConn3
  Phase Splitter1/RConn1 -- Variable Resistor/RConn1
  Phase Splitter1/LConn1 -- ~/RConn1
  Variable Resistor/LConn1 -- Simulink-PS Converter/RConn1 -- Variable Resistor2/LConn1 -- Variable Resistor1/LConn1
  Phase Splitter/LConn1 -- In/RConn1

== system IndustrialMicrogrid/MG1 Drilling Loads/Load Measurements1 ==
  Current and Voltage Sensor (Three-Phase)2 : ee_lib/Sensors & Transducers/Current and Voltage Sensor (Three-Phase)  vMeasurementType=ee.enum.vmeasurement.ll  outputUnit=ee.enum.unit.pu  SRated=1e6 A*V  VRated=microgrid.unitSubstationVoltage V  I_specify=off  I_priority=None  I=[0, 0, 0] A  I_nominal_specify=off  I_nominal_value=1  I_nominal_unit=A  V_specify=off  V_priority=None  V=[0, 0, 0] V  V_nominal_specify=off  V_nominal_value=1  V_nominal_unit=V
      settings: InternalSimscapePortConfiguration="{\"Bottom\":[],\"Left\":[{\"id\":\"N1\",\"label\":\"~1\",\"type\":\"foundation.electrical.three_phase\"}],\"Right\":[{\"id\":\"V_output\",\"label\":\"V\",\"type\":\"output\"},{\"id\":\"I_output\",\"label\":\"I\",\"type\":\"output\"},{\"id\":\"N2\",\"label\":\"~2\",\"type\":\"foundation.electrical.three_phase\"}],\"Top\":[]}"
  Low-Pass Filter (Discrete or Continuous)1 : eeGeneralControl/Low-Pass Filter (Discrete or Continuous)  K=1  T=0.02  B=inf  A=-inf  init_option=Inherited from block input  x0=0  Ts=Ts
  Low-Pass Filter (Discrete or Continuous)2 : eeGeneralControl/Low-Pass Filter (Discrete or Continuous)  K=1  T=0.02  B=inf  A=-inf  init_option=Inherited from block input  x0=0  Ts=Ts
  PS-Simulink Converter1 : nesl_utility_internal/PS-Simulink Converter  PhysicalDomain=network_engine_domain  SubClassName=ps_output  LeftPortType=input  RightPortType=output  PseudoPeriodic=off  Frequencies=[]  VectorFormat=1-D array  Unit=inherit  AffineConversion=off
  PS-Simulink Converter12 : nesl_utility_internal/PS-Simulink Converter  PhysicalDomain=network_engine_domain  SubClassName=ps_output  LeftPortType=input  RightPortType=output  PseudoPeriodic=off  Frequencies=[]  VectorFormat=1-D array  Unit=V  AffineConversion=off
  PS-Simulink Converter13 : nesl_utility_internal/PS-Simulink Converter  PhysicalDomain=network_engine_domain  SubClassName=ps_output  LeftPortType=input  RightPortType=output  PseudoPeriodic=off  Frequencies=[]  VectorFormat=1-D array  Unit=A  AffineConversion=off
  PS-Simulink Converter2 : nesl_utility_internal/PS-Simulink Converter  PhysicalDomain=network_engine_domain  SubClassName=ps_output  LeftPortType=input  RightPortType=output  PseudoPeriodic=off  Frequencies=[]  VectorFormat=1-D array  Unit=inherit  AffineConversion=off
  PS-Simulink Converter6 : nesl_utility_internal/PS-Simulink Converter  PhysicalDomain=network_engine_domain  SubClassName=ps_output  LeftPortType=input  RightPortType=output  PseudoPeriodic=off  Frequencies=[]  VectorFormat=1-D array  Unit=MW  AffineConversion=off
  PS-Simulink Converter7 : nesl_utility_internal/PS-Simulink Converter  PhysicalDomain=network_engine_domain  SubClassName=ps_output  LeftPortType=input  RightPortType=output  PseudoPeriodic=off  Frequencies=[]  VectorFormat=1-D array  Unit=MV*A  AffineConversion=off
  Power Sensor (Three-Phase)1 : ee_lib/Sensors & Transducers/Power Sensor (Three-Phase)  load_type=ee.enum.passive.type_balanced.balanced  f0=60 Hz  config=ee.enum.with_neutral.no  rho=1
      settings: InternalSimscapePortConfiguration="{\"Bottom\":[],\"Left\":[{\"id\":\"N1\",\"label\":\"~1\",\"type\":\"foundation.electrical.three_phase\"}],\"Right\":[{\"id\":\"N2\",\"label\":\"~2\",\"type\":\"foundation.electrical.three_phase\"}],\"Top\":[{\"id\":\"Pm\",\"label\":\"P\",\"type\":\"output\"},{\"id\":\"Qm\",\"label\":\"Q\",\"type\":\"output\"}]}"
  "Sinusoidal Measurement (PLL, Three-Phase)" : eeSinusoidalMeasurementV2/Sinusoidal Measurement (PLL, Three-Phase)  InputFilter=on  InputNormalization=off  Kp_LF=10  Ki_LF=200  F0=60  Theta0=0  Ts=Ts
      settings: LibrarySourceBlock=|
      | ee_sl_lib/Measurements/Sinusoidal Measurement
      | (PLL, Three-Phase)
  "Sinusoidal Measurement (PLL, Three-Phase)1" : eeSinusoidalMeasurementV2/Sinusoidal Measurement (PLL, Three-Phase)  InputFilter=on  InputNormalization=off  Kp_LF=10  Ki_LF=200  F0=60  Theta0=0  Ts=Ts
      settings: LibrarySourceBlock=|
      | ee_sl_lib/Measurements/Sinusoidal Measurement
      | (PLL, Three-Phase)
  Terminator{,1..3} (4 alike) : Terminator
  a2 : PMIOPort  Side=Left
  Conn2 : PMIOPort  Port=2  Side=Right
  Out Bus Element : Outport  PortName=mLoad  Element=activePower
  Out Bus Element1 : Outport  PortName=mLoad  Element=reactivePower
  Out Bus Element2 : Outport  PortName=mLoad  Element=voltage
  Out Bus Element3 : Outport  PortName=mLoad  Element=current
  Out Bus Element4 : Outport  PortName=mLoad  Element=voltageRMS
  Out Bus Element5 : Outport  PortName=mLoad  Element=currentRMS
  wires:
  PS-Simulink Converter12/1 -> Out Bus Element2/1
  PS-Simulink Converter13/1 -> Out Bus Element3/1
  PS-Simulink Converter7/1 -> Low-Pass Filter (Discrete or Continuous)2/1
  PS-Simulink Converter6/1 -> Low-Pass Filter (Discrete or Continuous)1/1
  PS-Simulink Converter1/1 -> "Sinusoidal Measurement (PLL, Three-Phase)"/1
  PS-Simulink Converter2/1 -> "Sinusoidal Measurement (PLL, Three-Phase)1"/1
  Low-Pass Filter (Discrete or Continuous)1/1 -> Out Bus Element/1
  Low-Pass Filter (Discrete or Continuous)2/1 -> Out Bus Element1/1
  "Sinusoidal Measurement (PLL, Three-Phase)1"/3 -> Out Bus Element5/1
  "Sinusoidal Measurement (PLL, Three-Phase)"/3 -> Out Bus Element4/1
  "Sinusoidal Measurement (PLL, Three-Phase)"/1 -> Terminator/1
  "Sinusoidal Measurement (PLL, Three-Phase)"/2 -> Terminator1/1
  "Sinusoidal Measurement (PLL, Three-Phase)1"/1 -> Terminator2/1
  "Sinusoidal Measurement (PLL, Three-Phase)1"/2 -> Terminator3/1
  connections:
  Power Sensor (Three-Phase)1/LConn3 -- PS-Simulink Converter7/LConn1
  Power Sensor (Three-Phase)1/LConn2 -- PS-Simulink Converter6/LConn1
  Current and Voltage Sensor (Three-Phase)2/RConn3 -- Conn2/RConn1
  a2/RConn1 -- Power Sensor (Three-Phase)1/LConn1
  Current and Voltage Sensor (Three-Phase)2/RConn1 -- PS-Simulink Converter12/LConn1 -- PS-Simulink Converter1/LConn1
  Current and Voltage Sensor (Three-Phase)2/RConn2 -- PS-Simulink Converter2/LConn1 -- PS-Simulink Converter13/LConn1
  Power Sensor (Three-Phase)1/RConn1 -- Current and Voltage Sensor (Three-Phase)2/LConn1
